simulink model "Buck_Converter_Open_Loop"  (R2015a)
settings: Solver=ode45  StartTime=0.0  StopTime=1  RelTol=1e-3
libraries: powerlib x9
settings Model: Creator=Koustubh  LastModifiedBy=Koustubh

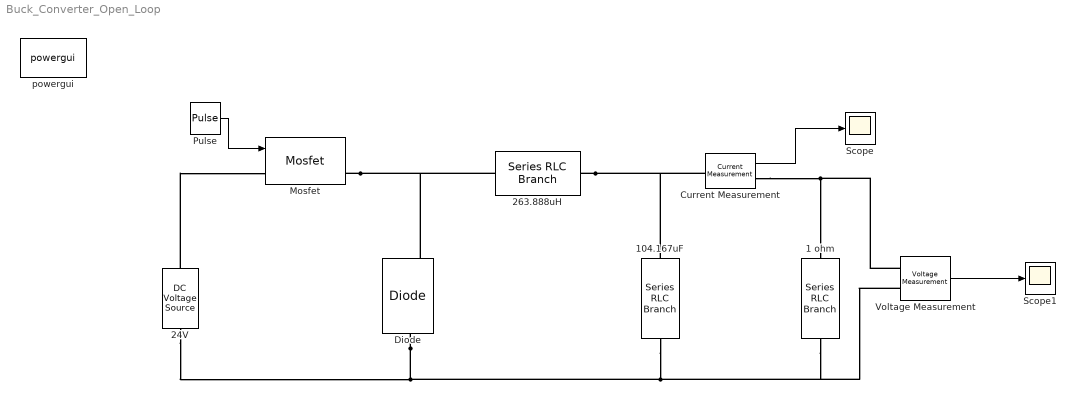
== system Buck_Converter_Open_Loop ==
  1 ohm : powerlib/Elements/Series RLC Branch  LConnTagsString=__new0  RConnTagsString=__new0  BranchType=R  Resistance=1  Inductance=1e-3  SetiL0=off  InitialCurrent=0  Capacitance=1e-6  Setx0=off  InitialVoltage=0  Measurements=None
  104.167uF : powerlib/Elements/Series RLC Branch  LConnTagsString=__new0  RConnTagsString=__new0  BranchType=C  Resistance=1  Inductance=1e-3  SetiL0=off  InitialCurrent=0  Capacitance=104.167e-6  Setx0=off  InitialVoltage=0  Measurements=None
  24V : powerlib/Electrical Sources/DC Voltage Source  Amplitude=24  Measurements=None
  263.888uH : powerlib/Elements/Series RLC Branch  LConnTagsString=__new0  RConnTagsString=__new0  BranchType=L  Resistance=1  Inductance=263.888e-6  SetiL0=off  InitialCurrent=0  Capacitance=1e-6  Setx0=off  InitialVoltage=0  Measurements=None
  Current Measurement : powerlib/Measurements/Current Measurement  PhasorSimulation=off  OutputType=Complex  PSBequivalent=0
  Diode : powerlib/Power Electronics/Diode  Ron=0.00001  Lon=0  Vf=0.01  IC=0  UseSnubber=off  Rs=500  Cs=250e-9  Measurements=on
  Mosfet : powerlib/Power Electronics/Mosfet  Ron=0.00001  Lon=0  Rd=0.00001  Vfd=0  IC=0  Rs=1e5  Cs=inf  Measurements=on
  "Pulse " : DiscretePulseGenerator  PulseType=Time based  Period=1/30000  PulseWidth=50
  Scope : Scope
  Scope1 : Scope
      settings: YMin=11.994  YMax=12.005
  Voltage Measurement : powerlib/Measurements/Voltage Measurement  PhasorSimulation=off  OutputType=Complex  PSBequivalent=0
  powergui : powerlib/powergui  Priority=1  SimulationMode=Continuous  SolverType=Tustin/Backward Euler (TBE)  SampleTime=50e-6  frequency=60  SPID=off  DisableSnubberDevices=off  DisableRonSwitches=off  DisableVfSwitches=off  SwTol=0  DisplayEquations=off  Interpol=off  methode=off  Ts=100  FunctionMessages=off  echomessages=off  HookPort=off  EnableUseOfTLC=off  x0status=blocks  frequencyindice=0  Pbase=100e6  ErrMax=1e-4  Iterations=50  UnitsV=kV  UnitsW=MW  buscounter=0  RestoreLinks=warning  ResistiveCurrentMeasurement=off  Frange=[0:2:500]  Ylog=off  Xlog=on  ShowGrid=off  save=off  variable=ZData  structure=ScopeData  ZoomFFT=off  StartTime=0.0  cycles=1  DisplayStyle=1  fundamental=60  FreqAxis=off  MaxFrequency=1000  frequencyindicesteady=1  RmsSteady=1  display=off
  wires:
  Current Measurement/1 -> Scope/1
  Voltage Measurement/1 -> Scope1/1
  "Pulse "/1 -> Mosfet/1
  connections:
  Mosfet/RConn1 -- 263.888uH/LConn1 -- Diode/RConn1
  263.888uH/RConn1 -- 104.167uF/LConn1 -- Current Measurement/LConn1
  Diode/LConn1 -- 24V/LConn1 -- 1 ohm/RConn1 -- Voltage Measurement/LConn2 -- 104.167uF/RConn1
  Voltage Measurement/LConn1 -- 1 ohm/LConn1 -- Current Measurement/RConn1
  24V/RConn1 -- Mosfet/LConn1
